simulink model "matlab_ppg_v3"  (R2018a)
settings: Solver=FixedStepAuto  StartTime=0.0  StopTime=60  RelTol=1e-3  EnableMultiTasking=on
libraries: dsparch4 x6, arduinolib x1, dspstat3 x1, dspxfrm3 x1
settings Model: SimulationMode=external  ExtModeTrigDuration=2  Creator=Na-Teng  LastModifiedBy=Na-Teng
settings OptimizationCC: EnhancedBackFolding=on  PassReuseOutputArgsAs=Individual arguments  MaxStackSize=64  OptimizeBlockOrder=speed  DifferentSizesBufferReuse=on  OptimizationCustomize=off
settings DebuggingCC: ParameterTunabilityLossMsg=error
settings HardwareCC: ProdBitPerInt=16  ProdBitPerPointer=16  ProdBitPerSizeT=16  ProdBitPerPtrDiffT=16  ProdLargestAtomicFloat=None  ProdWordSize=8  ProdHWDeviceType=Atmel->AVR
settings SFSimCC: MATLABDynamicMemAlloc=off
settings RTWCC: SystemTargetFile=ert.tlc  HardwareBoard=Arduino Mega 2560  TLCOptions=-aInlineSetEventsForThisBaseRateFcn=TLC_FALSE -aSuppressMultiTaskScheduler=TLC_FALSE -aRateBasedStepFcn=1  TemplateMakefile=ert_default_tmf  GenerateReport=on  Toolchain=Arduino AVR  BuildConfiguration=Faster Runs  IncludeHyperlinkInReport=on  LaunchReport=on  GenerateTraceInfo=on  GenerateTraceReport=on  GenerateTraceReportSl=on  GenerateTraceReportSf=on  GenerateTraceReportEml=on
settings CodeAppCC: ForceParamTrailComments=on  IgnoreCustomStorageClasses=off  OperatorAnnotations=on  SimulinkDataObjDesc=on  SFDataObjDesc=on  InsertBlockDesc=on
settings ERTTargetCC: SupportContinuousTime=on  SupportVariableSizeSignals=on

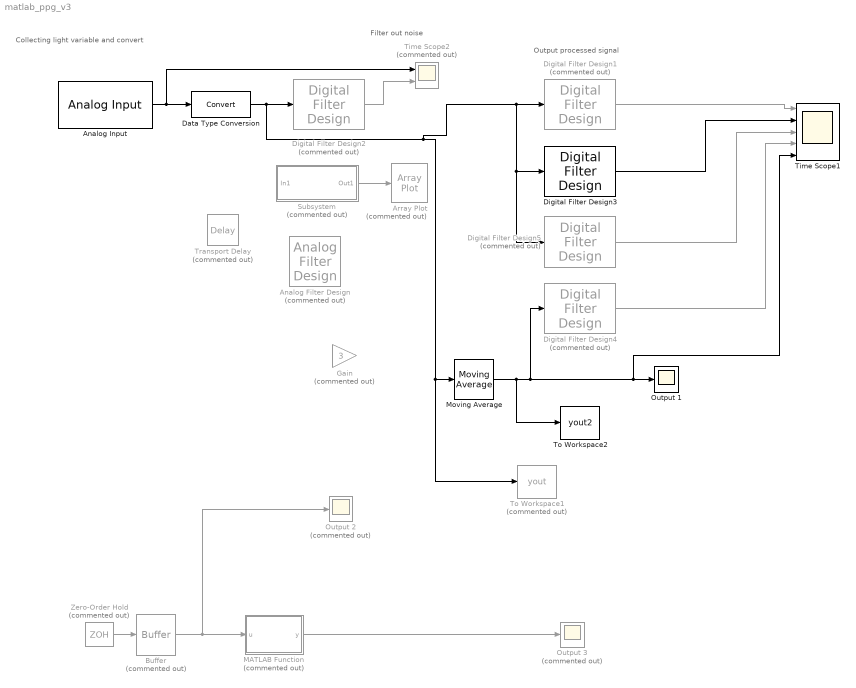
== system matlab_ppg_v3 ==
  note: Output processed signal
  note: Filter out noise
  note: Collecting light variable and convert
  Analog Filter Design : dsparch4/Analog Filter Design  Commented=on  method=Butterworth  filttype=Bandpass  N=8  Wlo=0.5  Whi=1.5  Rp=2  Rs=40
  Analog Input : arduinolib/Analog Input  pinNumber=4  ReadResultsOnly=off  ConversionTriggerSource=Software  ExternalTriggerType=uint32(0)  OutputDataType=uint16  EnableConversionCompleteNotify=off  EnableOuputStatus=off  SampleTime=0.001  blockPlatform=arduino
  Array Plot : ArrayPlot  Commented=on
  Buffer : Buffer  Commented=on  N=34  OutputFrames=off
  Data Type Conversion : DataTypeConversion
  Digital Filter Design{1..2,4..5} (4 alike) : dsparch4/Digital Filter Design  Commented=on  mwdsp_browser_bugfix_var=off
  Digital Filter Design3 : dsparch4/Digital Filter Design  mwdsp_browser_bugfix_var=off
  Gain : Gain  Commented=on  Gain=3
  MATLAB Function : MATLAB Function  Commented=on  TreatAsAtomicUnit=on
  Moving Average : dspstat3/Moving Average  Method=Sliding window  ForgettingFactorPort=off  SpecifyWindowLength=on  WindowLength=130  ForgettingFactor=0.9  SimulateUsing=Code generation
  Output 1 : Scope
  Output 2 : Scope  Commented=on
  Output 3 : Scope  Commented=on
  Subsystem : Subsystem  Commented=on
  Time Scope1 : Scope  NumInputPorts=5
  Time Scope2 : Scope  Commented=on  NumInputPorts=2
  To Workspace1 : ToWorkspace  Commented=on  VariableName=yout  SampleTime=-1
      settings: Save2DSignal=2-D array (concatenate along first dimension)
  To Workspace2 : ToWorkspace  VariableName=yout2  SaveFormat=Structure With Time  SampleTime=-1
      settings: Save2DSignal=2-D array (concatenate along first dimension)
  Transport Delay : TransportDelay  Commented=on
  Zero-Order Hold : ZeroOrderHold  Commented=on  SampleTime=-1
  wires:
  Analog Input/1 -> Time Scope2/1, Data Type Conversion/1
  Data Type Conversion/1 -> Digital Filter Design2/1, Digital Filter Design3/1, Digital Filter Design5/1, Digital Filter Design1/1, To Workspace1/1, Moving Average/1
  Digital Filter Design2/1 -> Time Scope2/2
  Subsystem/1(Out1) -> Array Plot/1
  MATLAB Function/1(y) -> Output 3/1
  Buffer/1 -> Output 2/1, MATLAB Function/1(u)
  Zero-Order Hold/1 -> Buffer/1
  Digital Filter Design1/1 -> Time Scope1/1
  Digital Filter Design3/1 -> Time Scope1/2
  Digital Filter Design5/1 -> Time Scope1/3
  Digital Filter Design4/1 -> Time Scope1/4
  Moving Average/1 -> To Workspace2/1, Digital Filter Design4/1, Time Scope1/5, Output 1/1

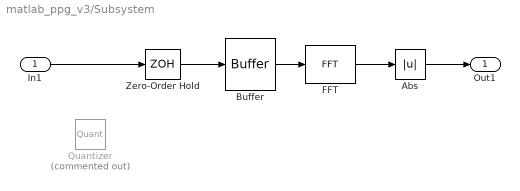
== system matlab_ppg_v3/Subsystem ==
  In1 : Inport
  Abs : Abs
  Buffer : Buffer  N=1536  OutputFrames=off
  FFT : dspxfrm3/FFT  FFTImplementation=Auto  CompMethod=Table lookup  TableOpt=NEW  TableOptActive=Speed  BitRevOrder=off  Normalize=off  InheritFFTLength=on  FFTLength=64  WrapInput=on  roundingMode=Floor  overflowMode=off  firstCoeffDataTypeStr=Inherit: Same word length as input  firstCoeffLastDataTypeStr=Inherit: Same word length as input  outputMin=[]  outputMax=[]
  Quantizer : Quantizer  Commented=on
  Zero-Order Hold : ZeroOrderHold  SampleTime=-1
  Out1 : Outport
  wires:
  Zero-Order Hold/1 -> Buffer/1
  Buffer/1 -> FFT/1
  FFT/1 -> Abs/1
  Abs/1 -> Out1/1
  In1/1 -> Zero-Order Hold/1

== matlab function matlab_ppg_v3/MATLAB Function ==
  data: u input; y output
function y = applyFilter(u)

y = sgolayfilt(u,1,3);
